simulink model "bexus_simple_pid_test"  (R2019a)
settings: Solver=FixedStepAuto  StartTime=0.0  StopTime=200  FixedStep=0.001  RelTol=1e-3
model workspace (MAT data in the model file):
  tau = 1.902274
values from neighbouring files (symbols this model uses):
  gyro_noise = ((deg2rad(0.15/60))^2)    [bexus_simple_pid_setup.m]
  motor_speed = 0.2272729091    [bexus_simple_pid_setup.m]
  random_seed = 23351    [bexus_simple_pid_setup.m]
libraries: simulink x11, simulink_extras x4, aerolibnav x1
settings Model: OrderedModelArguments=off  Creator=Jacek  LastModifiedBy=asmialek

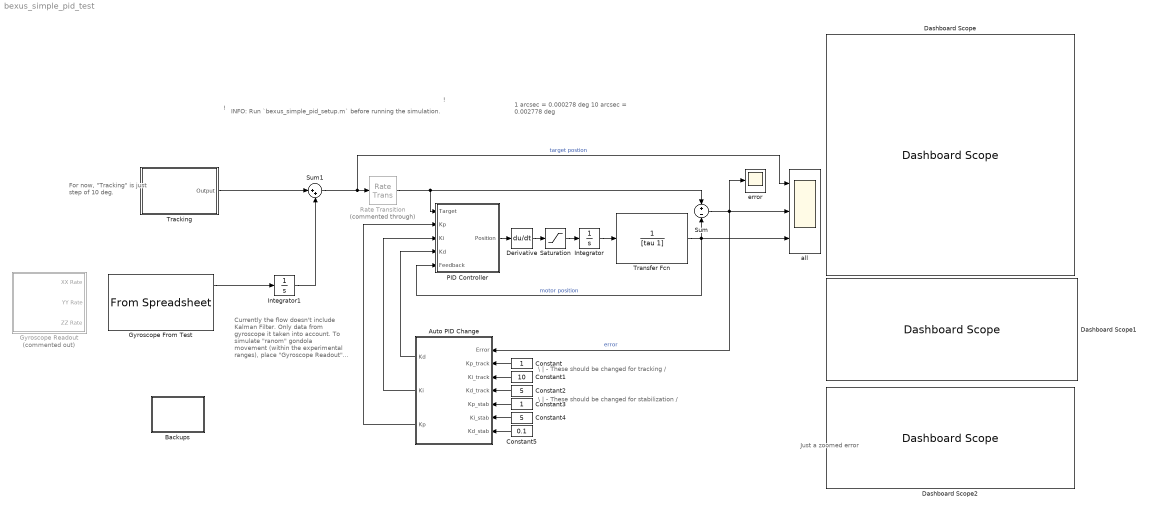
== system bexus_simple_pid_test ==
  note: !
  note: For now, "Tracking" is just step of 10 deg.
  note: \
      |  | - These should be changed for tracking
      | /
  note: 1 arcsec = 0.000278 deg
      | 10 arcsec = 0.002778 deg
  note: INFO: Run `bexus_simple_pid_setup.m` before running the simulation.
  note: Currently the flow doesn't include Kalman Filter. Only data from gyroscope it taken into account.
      |
      | To simulate "ranom" gondola movement (within the experimental ranges), place "Gyroscope Readout" subsystem in place of "Gyroscope From Test" block.
  note: Just a zoomed error
  note: \
      |  | - These should be changed for stabilization
      | /
  note: !
  Auto PID Change : Subsystem
  Backups : Subsystem
  Constant : Constant
  Constant1 : Constant  Value=10
  Constant2 : Constant  Value=5
  Constant3 : Constant
  Constant4 : Constant  Value=5
  Constant5 : Constant  Value=0.1
  Dashboard Scope : DashboardScope
  Dashboard Scope1 : DashboardScope  Ymin=-0.050000000000000003  Ymax=0.050000000000000003
  Dashboard Scope2 : DashboardScope  TimeSpan=30  Ymin=-0.010000000000000004  Ymax=0.010000000000000004  ScaleAtStop=off
  Derivative : Derivative
  Gyroscope From Test : FromSpreadsheet  FileName=/home/asmialek/Projects/BEXUS/irisc-control/gyro_data/gyro_16HzLP_new.xlsx
  Gyroscope Readout : Subsystem  Commented=on
  Integrator : Integrator
  Integrator1 : Integrator
  PID Controller : Subsystem
  Rate Transition : RateTransition  Commented=through  OutPortSampleTime=0.1
  Saturation : Saturate  UpperLimit=motor_speed  LowerLimit=-motor_speed
  Sum : Sum  Inputs=+|-
  Sum1 : Sum  Inputs=|++
  Tracking : Subsystem
  Transfer Fcn : TransferFcn  Denominator=[tau 1]
  all : Scope  NumInputPorts=3
  error : Scope
  wires:
  Rate Transition/1 -> PID Controller/1(Target), Sum/1
  PID Controller/1(Position) -> Derivative/1
  Sum/1 -> all/2, error/1, Auto PID Change/1(Error)  "error"
  Transfer Fcn/1 -> Sum/2, all/3, PID Controller/5(Feedback)  "motor position"
  Saturation/1 -> Integrator/1
  Auto PID Change/3(Kp) -> PID Controller/2(Kp)
  Auto PID Change/2(Ki) -> PID Controller/3(Ki)
  Auto PID Change/1(Kd) -> PID Controller/4(Kd)
  Derivative/1 -> Saturation/1
  Integrator/1 -> Transfer Fcn/1
  Tracking/1(Output) -> Sum1/1
  Sum1/1 -> all/1, Rate Transition/1  "target postion"
  Gyroscope From Test/1 -> Integrator1/1
  Integrator1/1 -> Sum1/2
  Constant/1 -> Auto PID Change/2(Kp_track)
  Constant1/1 -> Auto PID Change/3(Ki_track)
  Constant2/1 -> Auto PID Change/4(Kd_track)
  Constant3/1 -> Auto PID Change/5(Kp_stab)
  Constant4/1 -> Auto PID Change/6(Ki_stab)
  Constant5/1 -> Auto PID Change/7(Kd_stab)

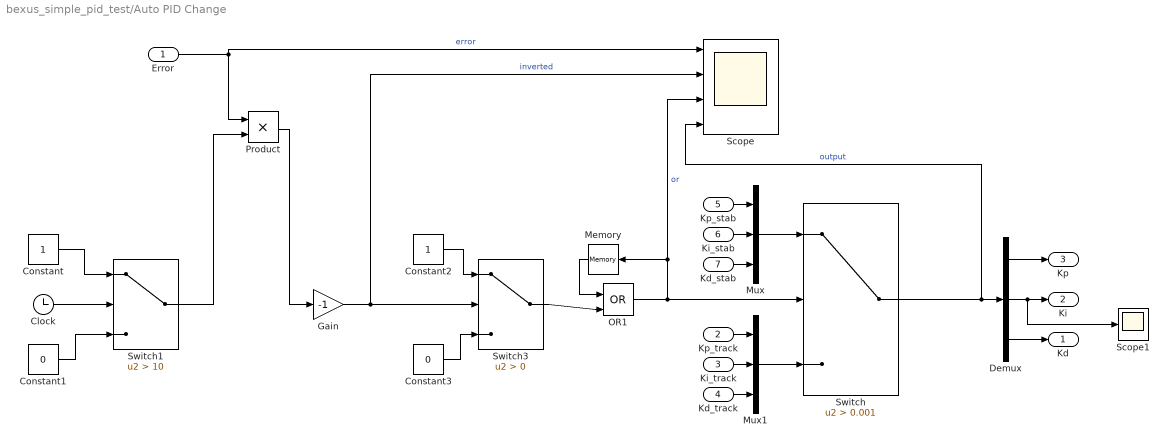
== system bexus_simple_pid_test/Auto PID Change ==
  Error : Inport
  Kp_track : Inport  Port=2
  Ki_track : Inport  Port=3
  Kd_track : Inport  Port=4
  Kp_stab : Inport  Port=5
  Ki_stab : Inport  Port=6
  Kd_stab : Inport  Port=7
  Clock : Clock
  Constant : Constant
  Constant1 : Constant  Value=0
  Constant2 : Constant
  Constant3 : Constant  Value=0
  Demux : Demux  Outputs=3
  Gain : Gain  Gain=-1
  Memory : Memory
  Mux : Mux  Inputs=3
  Mux1 : Mux  Inputs=3
  OR1 : Logic  Operator=OR  IconShape=distinctive  AllPortsSameDT=off  OutDataTypeStr=boolean
  Product : Product
  Scope : Scope  NumInputPorts=4
  Scope1 : Scope
  Switch : Switch  Criteria=u2 > Threshold  Threshold=0.001
  Switch1 : Switch  Criteria=u2 > Threshold  Threshold=10
  Switch3 : Switch  Criteria=u2 > Threshold
  Kd : Outport
  Ki : Outport  Port=2
  Kp : Outport  Port=3
  wires:
  Kp_stab/1 -> Mux/1
  Kp_track/1 -> Mux1/1
  Ki_track/1 -> Mux1/2
  Demux/2 -> Scope1/1, Ki/1
  Error/1 -> Product/1, Scope/1  "error"
  Demux/1 -> Kp/1
  Kd_stab/1 -> Mux/3
  Ki_stab/1 -> Mux/2
  Demux/3 -> Kd/1
  Kd_track/1 -> Mux1/3
  Mux/1 -> Switch/1
  Mux1/1 -> Switch/3
  Clock/1 -> Switch1/2
  Constant/1 -> Switch1/1
  Constant1/1 -> Switch1/3
  Product/1 -> Gain/1
  Switch1/1 -> Product/2
  Memory/1 -> OR1/1
  OR1/1 -> Memory/1, Scope/3, Switch/2  "or"
  Gain/1 -> Scope/2, Switch3/2  "inverted"
  Constant3/1 -> Switch3/3
  Constant2/1 -> Switch3/1
  Switch3/1 -> OR1/2
  Switch/1 -> Scope/4, Demux/1  "output"

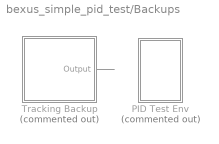
== system bexus_simple_pid_test/Backups ==
  PID Test Env : Subsystem  Commented=on
  Tracking Backup : Subsystem  Commented=on
  wires:
  Tracking Backup/1(Output) -> ?

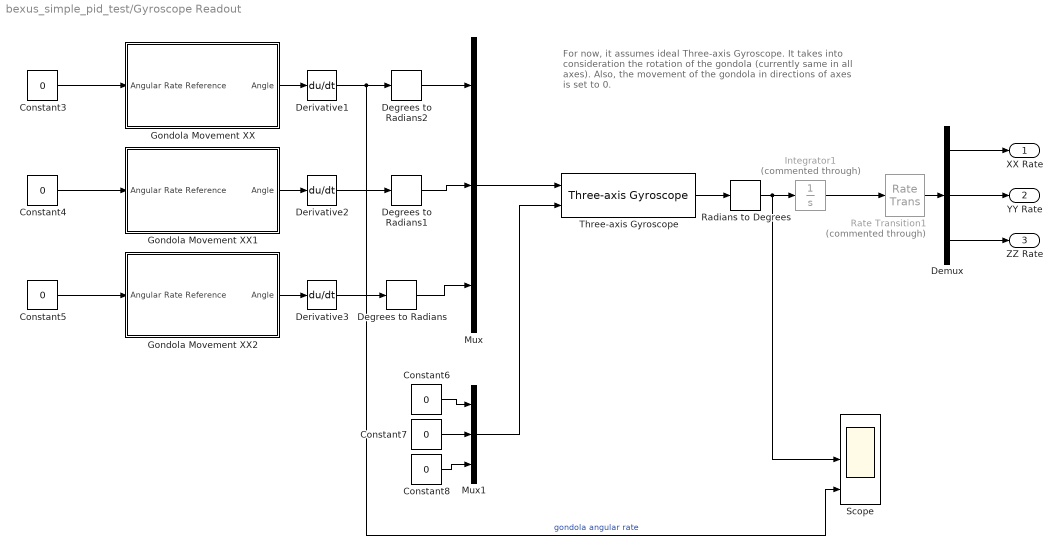
== system bexus_simple_pid_test/Gyroscope Readout ==
  note: For now, it assumes ideal Three-axis Gyroscope. It takes into consideration the rotation of the gondola (currently same in all axes). Also, the movement of the gondola in directions of axes is set to 0.
  Constant{3..8} (6 alike) : Constant  Value=0
  Degrees to Radians : simulink_extras/Transformations/Degrees to Radians
  Degrees to Radians1 : simulink_extras/Transformations/Degrees to Radians
  Degrees to Radians2 : simulink_extras/Transformations/Degrees to Radians
  Demux : Demux  Outputs=3
  Derivative1 : Derivative
  Derivative2 : Derivative
  Derivative3 : Derivative
  Gondola Movement XX : Subsystem
  Gondola Movement XX1 : Subsystem
  Gondola Movement XX2 : Subsystem
  Integrator1 : Integrator  Commented=through
  Mux : Mux  Inputs=3
  Mux1 : Mux  Inputs=3
  Radians to Degrees : simulink_extras/Transformations/Radians to Degrees
  Rate Transition1 : RateTransition  Commented=through  OutPortSampleTime=0.01
  Scope : Scope  NumInputPorts=3
  "Three-axis Gyroscope " : aerolibnav/Three-axis Gyroscope  dtype_g=off  w_g=190  z_g=0.707  g_sf_cc=[1 0 0; 0 1 0; 0 0 1]  g_bias=[0 0 0]  g_sen=[0 0 0]  g_Ts=-1  g_rand=off  g_seeds=[23093 23094 23095]  g_pow=[gyro_noise gyro_noise gyro_noise]  g_sat="[-inf  -inf  -inf  inf inf inf]"
      settings: SourceProductName=Aerospace Blockset  SourceProductBaseCode=AE
  XX Rate : Outport
  YY Rate : Outport  Port=2
  ZZ Rate : Outport  Port=3
  wires:
  Rate Transition1/1 -> Demux/1
  Constant3/1 -> Gondola Movement XX/1(Angular Rate Reference)
  Demux/2 -> YY Rate/1
  Constant8/1 -> Mux1/3
  Demux/1 -> XX Rate/1
  Demux/3 -> ZZ Rate/1
  Gondola Movement XX/1(Angle) -> Derivative1/1
  Gondola Movement XX2/1(Angle) -> Derivative3/1
  Gondola Movement XX1/1(Angle) -> Derivative2/1
  Constant5/1 -> Gondola Movement XX2/1(Angular Rate Reference)
  Mux1/1 -> "Three-axis Gyroscope "/2
  Mux/1 -> "Three-axis Gyroscope "/1
  Integrator1/1 -> Rate Transition1/1
  Constant6/1 -> Mux1/1
  Constant7/1 -> Mux1/2
  Constant4/1 -> Gondola Movement XX1/1(Angular Rate Reference)
  Radians to Degrees/1 -> Scope/2, Integrator1/1
  "Three-axis Gyroscope "/1 -> Radians to Degrees/1
  Degrees to Radians/1 -> Mux/3
  Derivative3/1 -> Degrees to Radians/1
  Derivative2/1 -> Degrees to Radians1/1
  Degrees to Radians1/1 -> Mux/2
  Derivative1/1 -> Scope/3, Degrees to Radians2/1  "gondola angular rate"
  Degrees to Radians2/1 -> Mux/1

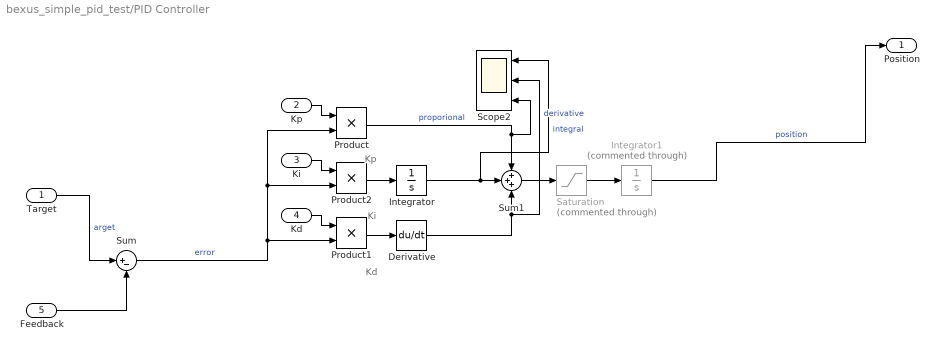
== system bexus_simple_pid_test/PID Controller ==
  note: Kd
  note: Ki
  note: Kp
  Target : Inport  SampleTime=0.1
  Kp : Inport  Port=2
  Ki : Inport  Port=3
  Kd : Inport  Port=4
  Feedback : Inport  Port=5
  Derivative : Derivative
  Integrator : Integrator
  Integrator1 : Integrator  Commented=through  InitialCondition=1
  Product : Product
  Product1 : Product
  Product2 : Product
  Saturation : Saturate  Commented=through  UpperLimit=0.05  LowerLimit=-0.05
  Scope2 : Scope  NumInputPorts=3
  Sum : Sum  Inputs=|+-
  Sum1 : Sum  Inputs=+++
  Position : Outport
  wires:
  Product2/1 -> Integrator/1
  Sum/1 -> Product1/2, Product2/2, Product/2  "error"
  Integrator1/1 -> Position/1  "position"
  Product/1 -> Sum1/1, Scope2/3  "proporional"
  Derivative/1 -> Scope2/2, Sum1/3  "derivative"
  Integrator/1 -> Scope2/1, Sum1/2  "integral"
  Sum1/1 -> Saturation/1
  Product1/1 -> Derivative/1
  Saturation/1 -> Integrator1/1
  Target/1 -> Sum/1  "arget"
  Feedback/1 -> Sum/2
  Ki/1 -> Product2/1
  Kd/1 -> Product1/1
  Kp/1 -> Product/1

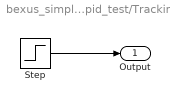
== system bexus_simple_pid_test/Tracking ==
  Step : Step  Time=5  After=10  SampleTime=0
  Output : Outport
  wires:
  Step/1 -> Output/1

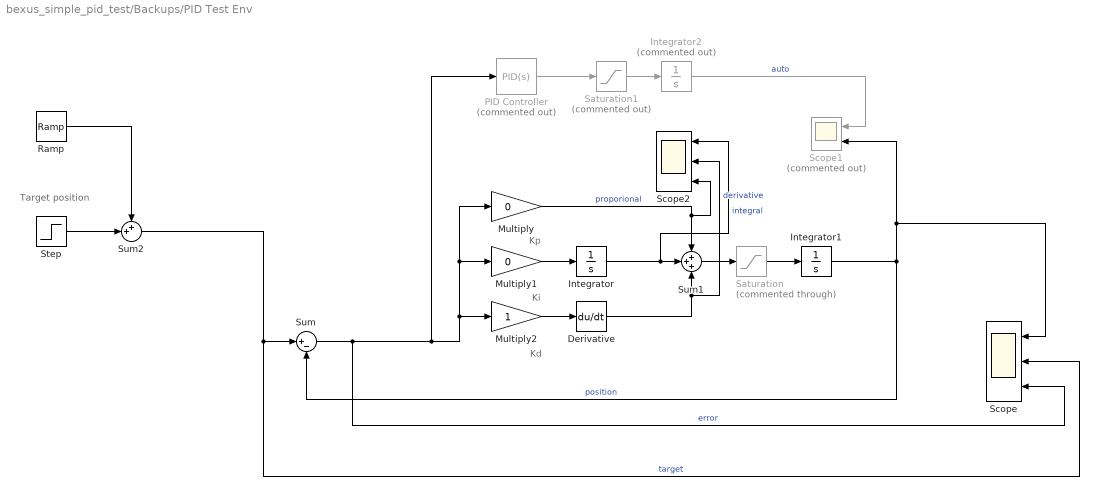
== system bexus_simple_pid_test/Backups/PID Test Env ==
  note: Kd
  note: Ki
  note: Kp
  note: Target position
  Derivative : Derivative
  Integrator : Integrator
  Integrator1 : Integrator  InitialCondition=1
  Integrator2 : Integrator  Commented=on  InitialCondition=1
  Multiply : Gain  Gain=0
  Multiply1 : Gain  Gain=0
  Multiply2 : Gain
  PID Controller : simulink/Continuous/PID Controller  Commented=on  Controller=PID  Form=Parallel  TimeDomain=Continuous-time  SampleTime=-1  IntegratorMethod=Forward Euler  FilterMethod=Forward Euler  ControllerParametersSource=internal  P=1  I=0.005  D=1  UseFilter=on  N=100  TunerSelectOption=Transfer Function Based (PID Tuner App)  InitialConditionSource=internal  InitialConditionForIntegrator=0  InitialConditionForFilter=0  DifferentiatorICPrevScaledInput=0  ExternalReset=none  TrackingMode=off  Kt=1  LimitOutput=off  UpperSaturationLimit=inf  LowerSaturationLimit=-inf  LinearizeAsGain=on  AntiWindupMode=none  Kb=1  POutMin=[]  POutMax=[]  IOutMin=[]  IOutMax=[]  DOutMin=[]  DOutMax=[]  NOutMin=[]  NOutMax=[]  SumOutMin=[]  SumOutMax=[]  SaturationOutMin=[]  SaturationOutMax=[]  PParamMin=[]  PParamMax=[]  IParamMin=[]  IParamMax=[]  DParamMin=[]  DParamMax=[]  NParamMin=[]  NParamMax=[]  KbParamMin=[]  KbParamMax=[]  KtParamMin=[]  KtParamMax=[]  KbOutMin=[]  KbOutMax=[]  KtOutMin=[]  KtOutMax=[]  IntegratorOutMin=[]  IntegratorOutMax=[]  FilterOutMin=[]  FilterOutMax=[]  SumI1OutMin=[]  SumI1OutMax=[]  SumI2OutMin=[]  SumI2OutMax=[]  SumI3OutMin=[]  SumI3OutMax=[]  SumI4OutMin=[]  SumI4OutMax=[]  SumDOutMin=[]  SumDOutMax=[]  DifferentiatorOutMin=[]  DifferentiatorOutMax=[]  FilterDiffOutCoefMin=[]  FilterDiffOutCoefMax=[]  ReciprocalOutMin=[]  ReciprocalOutMax=[]  SumDenOutMin=[]  SumDenOutMax=[]  SumNumOutMin=[]  SumNumOutMax=[]  DivideOutMin=[]  DivideOutMax=[]  IntegratorContinuousStateAttributes=''  IntegratorStateMustResolveToSignalObject=off  IntegratorRTWStateStorageClass=Auto  FilterContinuousStateAttributes=''  FilterStateMustResolveToSignalObject=off  FilterRTWStateStorageClass=Auto  ParallelPVariant=InternalParameters  IdealPVariant=Disabled  IVariant=InternalParameters  DVariant=InternalParameters  IntegratorVariant=Continuous  SatVariant=Disabled  AWVariant=Passthrough  PCopyVariant=Disabled  TRVariant=Disabled  FdbkBlocksVariant=Forward  IdealPFdbkVariant=Disabled  SatFdbkVariant=Disabled  DerivativeFilterVariant=ContFilter  NVariant=InternalParameters  NCopyVariant=Disabled  FilterICVariant=InternalICsFilter  IntegratorICVariant=InternalICs  ExternalResetVariant=Disabled  TRSumVariant=Passthrough  SumFdbkVariant=Disabled  SumVariant=Sum_PID
  Ramp : simulink/Sources/Ramp  slope=0.1  start=0  InitialOutput=0
  Saturation : Saturate  Commented=through  UpperLimit=0.05  LowerLimit=-0.05
  Saturation1 : Saturate  Commented=on  UpperLimit=0.05  LowerLimit=-0.05
  Scope : Scope  NumInputPorts=3
  Scope1 : Scope  Commented=on  NumInputPorts=2
  Scope2 : Scope  NumInputPorts=3
  Step : Step  Time=0  After=0.5  SampleTime=0
  Sum : Sum  Inputs=|+-
  Sum1 : Sum  Inputs=+++
  Sum2 : Sum  Inputs=++|
  wires:
  Multiply1/1 -> Integrator/1
  Sum/1 -> Scope/3, PID Controller/1, Multiply2/1, Multiply/1, Multiply1/1  "error"
  Integrator2/1 -> Scope1/1  "auto"
  Step/1 -> Sum2/2
  Sum2/1 -> Scope/2, Sum/1  "target"
  Integrator1/1 -> Sum/2, Scope1/2, Scope/1  "position"
  Multiply/1 -> Sum1/1, Scope2/3  "proporional"
  Derivative/1 -> Scope2/2, Sum1/3  "derivative"
  PID Controller/1 -> Saturation1/1
  Integrator/1 -> Scope2/1, Sum1/2  "integral"
  Sum1/1 -> Saturation/1
  Multiply2/1 -> Derivative/1
  Saturation/1 -> Integrator1/1
  Saturation1/1 -> Integrator2/1
  Ramp/1 -> Sum2/1

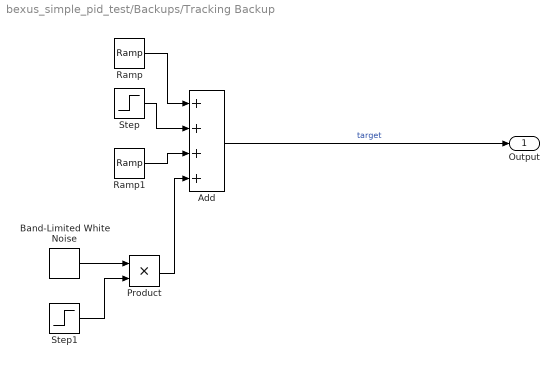
== system bexus_simple_pid_test/Backups/Tracking Backup ==
  Add : Sum  Inputs=++++
  Band-Limited White Noise : simulink/Sources/Band-Limited White Noise  Cov=[0.1]  Ts=0.5  seed=[23341]
  Product : Product
  Ramp : simulink/Sources/Ramp  slope=0.1  start=0  InitialOutput=0
  Ramp1 : simulink/Sources/Ramp  slope=-0.1  start=10  InitialOutput=0
  Step : Step  Time=20  After=0.5  SampleTime=0
  Step1 : Step  Time=40  After=0.01  SampleTime=0
  Output : Outport
  wires:
  Step1/1 -> Product/2
  Product/1 -> Add/4
  Ramp/1 -> Add/1
  Ramp1/1 -> Add/3
  Band-Limited White Noise/1 -> Product/1
  Step/1 -> Add/2
  Add/1 -> Output/1  "target"

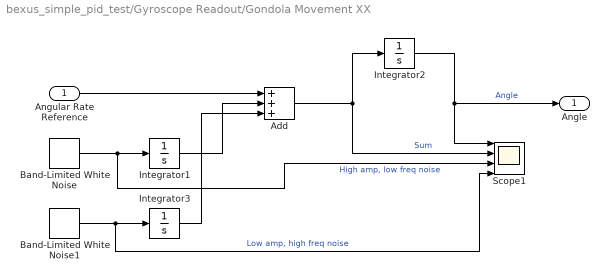
== system bexus_simple_pid_test/Gyroscope Readout/Gondola Movement XX ==
  Angular Rate Reference : Inport
  Add : Sum  Inputs=+++
  Band-Limited White Noise : simulink/Sources/Band-Limited White Noise  Cov=h_amp_noise_power  Ts=10  seed=[random_seed]
  Band-Limited White Noise1 : simulink/Sources/Band-Limited White Noise  Cov=l_amp_noise_power  Ts=1  seed=[random_seed]
  Integrator1 : Integrator
  Integrator2 : Integrator
  Integrator3 : Integrator
  Scope1 : Scope  NumInputPorts=4
  Angle : Outport
  wires:
  Integrator1/1 -> Add/2
  Band-Limited White Noise1/1 -> Scope1/4, Integrator3/1  "Low amp, high freq noise"
  Add/1 -> Integrator2/1, Scope1/2  "Sum"
  Band-Limited White Noise/1 -> Scope1/3, Integrator1/1  "High amp, low freq noise"
  Integrator3/1 -> Add/3
  Integrator2/1 -> Angle/1, Scope1/1  "Angle"
  Angular Rate Reference/1 -> Add/1

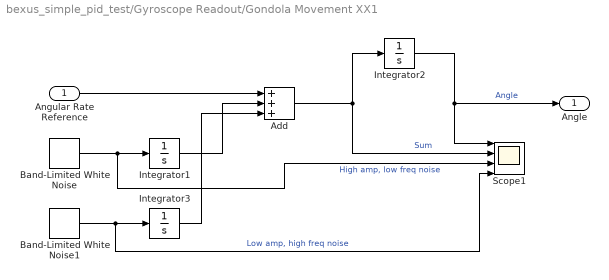
== system bexus_simple_pid_test/Gyroscope Readout/Gondola Movement XX1 ==
  Angular Rate Reference : Inport
  Add : Sum  Inputs=+++
  Band-Limited White Noise : simulink/Sources/Band-Limited White Noise  Cov=h_amp_noise_power  Ts=10  seed=[random_seed]
  Band-Limited White Noise1 : simulink/Sources/Band-Limited White Noise  Cov=l_amp_noise_power  Ts=1  seed=[random_seed]
  Integrator1 : Integrator
  Integrator2 : Integrator
  Integrator3 : Integrator
  Scope1 : Scope  NumInputPorts=4
  Angle : Outport
  wires:
  Integrator1/1 -> Add/2
  Band-Limited White Noise1/1 -> Scope1/4, Integrator3/1  "Low amp, high freq noise"
  Add/1 -> Integrator2/1, Scope1/2  "Sum"
  Band-Limited White Noise/1 -> Scope1/3, Integrator1/1  "High amp, low freq noise"
  Integrator3/1 -> Add/3
  Integrator2/1 -> Angle/1, Scope1/1  "Angle"
  Angular Rate Reference/1 -> Add/1

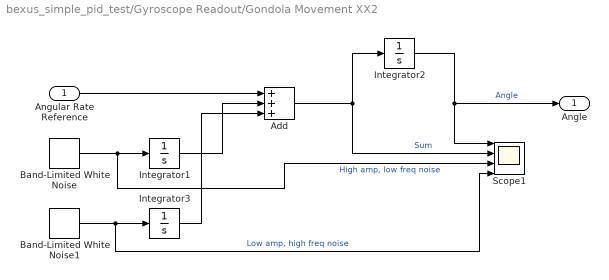
== system bexus_simple_pid_test/Gyroscope Readout/Gondola Movement XX2 ==
  Angular Rate Reference : Inport
  Add : Sum  Inputs=+++
  Band-Limited White Noise : simulink/Sources/Band-Limited White Noise  Cov=h_amp_noise_power  Ts=10  seed=[random_seed]
  Band-Limited White Noise1 : simulink/Sources/Band-Limited White Noise  Cov=l_amp_noise_power  Ts=1  seed=[random_seed]
  Integrator1 : Integrator
  Integrator2 : Integrator
  Integrator3 : Integrator
  Scope1 : Scope  NumInputPorts=4
  Angle : Outport
  wires:
  Integrator1/1 -> Add/2
  Band-Limited White Noise1/1 -> Scope1/4, Integrator3/1  "Low amp, high freq noise"
  Add/1 -> Integrator2/1, Scope1/2  "Sum"
  Band-Limited White Noise/1 -> Scope1/3, Integrator1/1  "High amp, low freq noise"
  Integrator3/1 -> Add/3
  Integrator2/1 -> Angle/1, Scope1/1  "Angle"
  Angular Rate Reference/1 -> Add/1
